simulink model "SAS_GeometryBlock"  (R2026a)
settings: Solver=VariableStepAuto  StopTime=5
undefined symbols (not defined in the file): delta, Q, theta, vel
libraries: simulink x1, slpidlib x1
settings Model: Creator=piotr  LastModifiedBy=piotr

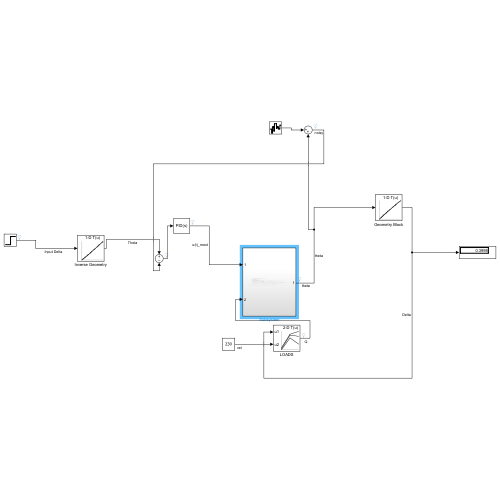
[thumbnail: Simulink's stored preview of the top-level diagram]
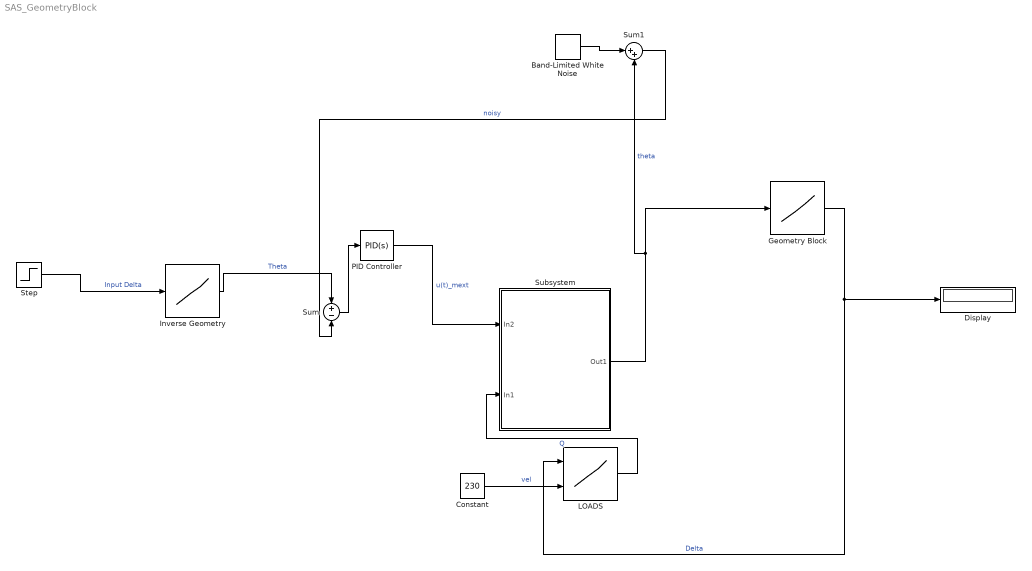
== system SAS_GeometryBlock ==
  Band-Limited White Noise : simulink/Sources/Band-Limited White Noise  Cov=[0.0000001]  Ts=0.1  seed=[23341]
  Constant : Constant  Value=230
  Display : Display
  Geometry Block : Lookup_n-D  NumberOfTableDimensions=1  BreakpointsForDimension1=theta  Table=delta  InternalRulePriority=Speed  RndMeth=Simplest
  Inverse Geometry : Lookup_n-D  NumberOfTableDimensions=1  BreakpointsForDimension1=delta  Table=theta  InternalRulePriority=Speed  RndMeth=Simplest
  LOADS : Lookup_n-D  BreakpointsForDimension1=delta  BreakpointsForDimension2=vel  Table=Q  InternalRulePriority=Speed  RndMeth=Simplest
      settings: InputPortMap=u0,u1
  PID Controller : slpidlib/PID Controller  Controller=PID  Form=Parallel  TimeDomain=Continuous-time  UseExternalTs=off  SampleTime=-1  IntegratorMethod=Forward Euler  FilterMethod=Forward Euler  ControllerParametersSource=internal  P=7481856804.6589  I=6415899462009.41  UseKiTs=off  D=2142362.37266913  UseExternalDerivativeSource=off  N=99977.4022895171  UseFilter=on  TunerSelectOption=Transfer Function Based (PID Tuner App)  InitialConditionSource=internal  InitialConditionForIntegrator=0  InitialConditionForFilter=0  DifferentiatorICPrevScaledInput=0  ExternalReset=none  TrackingMode=off  Kt=1  LimitOutput=off  SatLimitsSource=internal  UpperSaturationLimit=inf  LowerSaturationLimit=-inf  LinearizeAsGain=on  AntiWindupMode=none  Kb=1  LimitIntegrator=off  UpperIntegratorSaturationLimit=inf  LowerIntegratorSaturationLimit=-inf  POutMin=[]  POutMax=[]  IOutMin=[]  IOutMax=[]  DOutMin=[]  DOutMax=[]  NOutMin=[]  NOutMax=[]  SumOutMin=[]  SumOutMax=[]  SaturationOutMin=[]  SaturationOutMax=[]  PParamMin=[]  PParamMax=[]  IParamMin=[]  IParamMax=[]  DParamMin=[]  DParamMax=[]  NParamMin=[]  NParamMax=[]  KbParamMin=[]  KbParamMax=[]  KtParamMin=[]  KtParamMax=[]  KbOutMin=[]  KbOutMax=[]  KtOutMin=[]  KtOutMax=[]  IntegratorOutMin=[]  IntegratorOutMax=[]  FilterOutMin=[]  FilterOutMax=[]  SumI1OutMin=[]  SumI1OutMax=[]  SumI2OutMin=[]  SumI2OutMax=[]  SumI3OutMin=[]  SumI3OutMax=[]  SumI4OutMin=[]  SumI4OutMax=[]  SumDOutMin=[]  SumDOutMax=[]  DifferentiatorOutMin=[]  DifferentiatorOutMax=[]  FilterDiffOutCoefMin=[]  FilterDiffOutCoefMax=[]  ReciprocalOutMin=[]  ReciprocalOutMax=[]  SumDenOutMin=[]  SumDenOutMax=[]  SumNumOutMin=[]  SumNumOutMax=[]  DivideOutMin=[]  DivideOutMax=[]  UdiffTsProdOutMin=[]  UdiffTsProdOutMax=[]  NTsProdOutMin=[]  NTsProdOutMax=[]  UintegralTsProdOutMin=[]  UintegralTsProdOutMax=[]  UngainTsProdOutMin=[]  UngainTsProdOutMax=[]  ClampingZeroOutDataTypeStr=Inherit: Inherit via back propagation  ClampingZeroOutMin=[]  ClampingZeroOutMax=[]  FilterDenConstantOutDataTypeStr=Inherit: Inherit via back propagation  FilterDenConstantOutMin=[]  FilterDenConstantOutMax=[]  PCopyOutDataTypeStr=Inherit: Inherit via back propagation  PCopyOutMin=[]  PCopyOutMax=[]  NCopyOutDataTypeStr=Inherit: Inherit via back propagation  NCopyOutMin=[]  NCopyOutMax=[]  IntegratorContinuousStateAttributes=''  IntegratorStateMustResolveToSignalObject=off  IntegratorRTWStateStorageClass=Auto  FilterContinuousStateAttributes=''  FilterStateMustResolveToSignalObject=off  FilterRTWStateStorageClass=Auto  ParallelPVariant=InternalParameters  IdealPVariant=Disabled  IVariant=InternalParameters  DVariant=InternalParameters  IntegratorVariant=Continuous  SatVariant=Disabled  AWVariant=Passthrough  PCopyVariant=Disabled  TRVariant=Disabled  FdbkBlocksVariant=Forward  IdealPFdbkVariant=Disabled  SatFdbkVariant=Disabled  DerivativeFilterVariant=ContFilter  NVariant=InternalParameters  NCopyVariant=Disabled  FilterICVariant=InternalICsFilter  IntegratorICVariant=InternalICs  ExternalResetVariant=Disabled  TRSumVariant=Passthrough  SumFdbkVariant=Disabled  SumVariant=Sum_PID  TsampFilterVariant=InternalTs  TsampNgainVariant=Passthrough  TsampIntegralVariant=Disabled_SignalSpec  ExternalSaturationOutDataTypeStr=Inherit: Same as second input  DerivativeSourceVariant=ErrorSignal  PreIntVariant=InternalPreInt
  Step : Step  Time=0.001  FinalValue=0.4  SampleTime=0
  Subsystem : Subsystem
  Sum : Sum  Inputs=+-
  Sum1 : Sum  Inputs=|++
  wires:
  Inverse Geometry/1 -> Sum/1  "Theta"
  Step/1 -> Inverse Geometry/1  "Input Delta"
  Geometry Block/1 -> LOADS/1, Display/1  "Delta"
  LOADS/1 -> Subsystem/2(In1)  "Q"
  Constant/1 -> LOADS/2  "vel"
  Subsystem/1(Out1) -> Sum1/2, Geometry Block/1  "theta"
  Sum/1 -> PID Controller/1
  PID Controller/1 -> Subsystem/1(In2)  "u(t)_mext"
  Band-Limited White Noise/1 -> Sum1/1
  Sum1/1 -> Sum/2  "noisy"

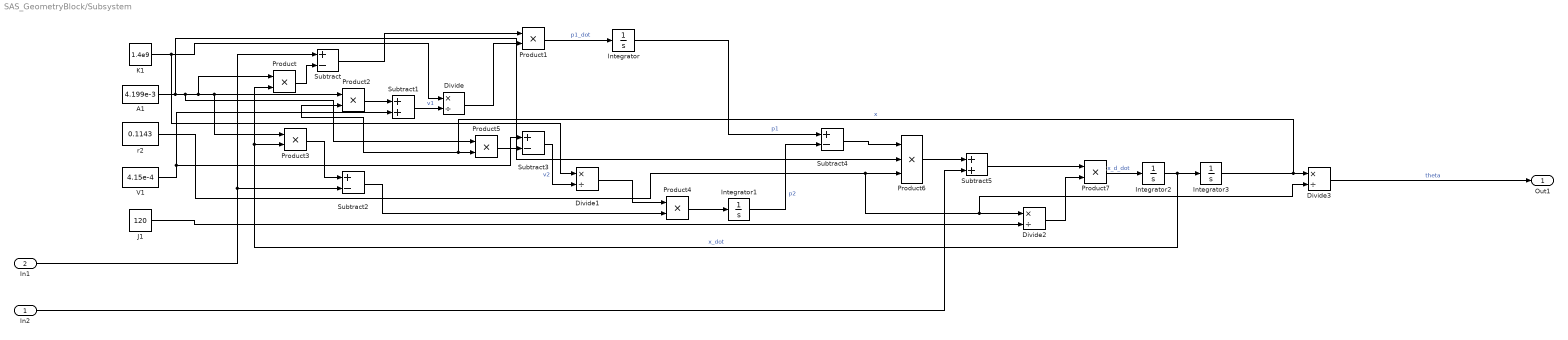
== system SAS_GeometryBlock/Subsystem ==
  In2 : Inport
  In1 : Inport  Port=2
  A1 : Constant  Value=4.199e-3
  Divide{,1..3} (4 alike) : Product  Inputs=*/
  Integrator : Integrator  InitialCondition=1e7  LimitOutput=on  UpperSaturationLimit=1.38e7  LowerSaturationLimit=0
  Integrator1 : Integrator  InitialCondition=1e7  LimitOutput=on  UpperSaturationLimit=1.38e7  LowerSaturationLimit=0
  Integrator2 : Integrator
  Integrator3 : Integrator  LimitOutput=on  UpperSaturationLimit=0.09  LowerSaturationLimit=-0.09
  J1 : Constant  Value=120
  K1 : Constant  Value=1.4e9
  Product{,1..5,7} (7 alike) : Product
  Product6 : Product  Inputs=3
  Subtract{,2..4} (4 alike) : Sum  Inputs=+-
  Subtract1 : Sum
  Subtract5 : Sum
  V1 : Constant  Value=4.15e-4
  r2 : Constant  Value=0.1143
  Out1 : Outport
  wires:
  Integrator3/1 -> Product2/2, Product5/2, Divide3/1  "x"
  Divide2/1 -> Product7/2
  Subtract1/1 -> Divide/2  "v1"
  Product2/1 -> Subtract1/1
  J1/1 -> Divide2/2
  In1/1 -> Subtract/1, Subtract2/2
  r2/1 -> Divide3/2, Divide2/1, Product6/3
  Divide3/1 -> Out1/1  "theta"
  V1/1 -> Subtract1/2, Subtract3/1
  Integrator2/1 -> Product3/2, Product/2, Integrator3/1  "x_dot"
  A1/1 -> Product6/2, Product5/1, Product3/1, Product2/1, Product/1
  Divide/1 -> Product1/2
  Product5/1 -> Subtract3/2
  Product/1 -> Subtract/2
  Integrator/1 -> Subtract4/1  "p1"
  Divide1/1 -> Product4/1
  Subtract4/1 -> Product6/1
  Subtract3/1 -> Divide1/2  "v2"
  Subtract/1 -> Product1/1
  Product1/1 -> Integrator/1  "p1_dot"
  Integrator1/1 -> Subtract4/2  "p2"
  K1/1 -> Divide1/1, Divide/1
  Product6/1 -> Subtract5/1
  Product3/1 -> Subtract2/1
  Product7/1 -> Integrator2/1  "x_d_dot"
  Subtract5/1 -> Product7/1
  Subtract2/1 -> Product4/2
  In2/1 -> Subtract5/2
  Product4/1 -> Integrator1/1
